simulink library "PowerFlowLib"  (Simulink 8.1)
settings: Solver=ode45  StartTime=0.0  StopTime=10.0  RelTol=1e-3
undefined symbols (not defined in the file or in its folder): Air, AirProp, C, F1, F2, Fanmap, Fld1, Fld2, Fluid, fueltankdata, HydProp, HydraulicLoad, IBFD_exc, L, LoadFluidProps, magnitude, MSSN, n_alghts, PumpProp, pwr_alghts, R_fd_exc, Rcore, Ts, VBFD_exc
libraries: PowerFlowLib x35, simulink x19, powerlib_extras x2, dspstat3 x2
(part 7 of 12)

== system PowerFlowLib/Energy & Power Systems/Electrical/Loads/Constant Current Load ==
  I_rms : Inport
  P.F. : Inport  Port=2
  Vabc : Inport  Port=3
  Eta1 : Inport  Port=4
  Constant : Constant  Value=[0 -2*pi/3 2*pi/3]
  Demux : Demux  Outputs=3
  Fcn1 : Fcn  Expr=(u(1)<=1)*(1-u(1))
  Math Function : Math  Operator=square  SaturateOnIntegerOverflow=on
  Mean Value : powerlib_extras/Measurements/Mean Value  Period=1/60
  Product{,1..6} (7 alike) : Product  RndMeth=Zero
  Sqrt : Sqrt  SaturateOnIntegerOverflow=on
  Sum : Sum  Inputs=|+-
  Sum1 : Sum
  Trigonometric Function : Trigonometry  Operator=acos
  Trigonometric Function1 : Trigonometry
  Trigonometric Function2 : Trigonometry  Operator=atan2
  Trigonometric Function3 : Trigonometry  Operator=cos
  Trigonometric Function4 : Trigonometry
  abc to qd0 : Subsystem
  iabc : Outport
  P : Outport  Port=2
  P_loss1 : Outport  Port=3
  Q : Outport  Port=4
  wires:
  Math Function/1 -> Mean Value/1
  Mean Value/1 -> Sqrt/1
  Sqrt/1 -> Product4/2, Product6/2  "RMS"
  I_rms/1 -> Product/1, Product1/1
  P.F./1 -> Product/2, Trigonometric Function/1
  Trigonometric Function/1 -> Trigonometric Function1/1
  Trigonometric Function1/1 -> Product1/2
  Product/1 -> Product2/1, Product6/1
  Vabc/1 -> Demux/1
  Demux/1 -> abc to qd0/1(V_a), Math Function/1
  Demux/2 -> abc to qd0/2(V_b)
  Demux/3 -> abc to qd0/3(V_c)
  Trigonometric Function3/1 -> Product2/2
  Trigonometric Function4/1 -> Product3/2
  Trigonometric Function2/1 -> Sum/1
  Constant/1 -> Sum/2
  Sum/1 -> Trigonometric Function3/1, Trigonometric Function4/1
  Product2/1 -> Sum1/1
  Product3/1 -> Sum1/2
  Sum1/1 -> iabc/1
  abc to qd0/2(V_d) -> Trigonometric Function2/1
  abc to qd0/1(V_q) -> Trigonometric Function2/2
  Product1/1 -> Product3/1, Product4/1
  Eta1/1 -> Fcn1/1
  Product5/1 -> P_loss1/1
  Product6/1 -> P/1, Product5/1
  Product4/1 -> Q/1
  Fcn1/1 -> Product5/2

== system PowerFlowLib/Energy & Power Systems/Electrical/Loads/Constant Power Load ==
  S : Inport
  P.F. : Inport  Port=2
  Vabc : Inport  Port=3
  Eta : Inport  Port=4
  Constant : Constant  Value=[0 -2*pi/3 2*pi/3]
  Demux : Demux  Outputs=3
  Fcn : Fcn  Expr=u(1)/(u(3)+0.01)
  Fcn1 : Fcn  Expr=u(2)/(u(3)+0.01)
  Fcn2 : Fcn  Expr=(u(1)<=1)*(1-u(1))
  Math Function : Math  Operator=square  SaturateOnIntegerOverflow=on
  Mean Value : powerlib_extras/Measurements/Mean Value  Period=1/60
  Mux : Mux  Inputs=3
  Product{,1..4} (5 alike) : Product  RndMeth=Zero
  Scope : Scope
      settings: TimeRange=auto  MaxDataPoints=5000  SaveToWorkspace=off  SaveName=ScopeData  YMin=-10  YMax=10  SampleTime=-1
  Sqrt : Sqrt  SaturateOnIntegerOverflow=on
  Sum : Sum  Inputs=|+-
  Sum1 : Sum
  Trigonometric Function : Trigonometry  Operator=acos
  Trigonometric Function1 : Trigonometry
  Trigonometric Function2 : Trigonometry  Operator=atan2
  Trigonometric Function3 : Trigonometry  Operator=cos
  Trigonometric Function4 : Trigonometry
  abc to qd0 : Subsystem
  iabc : Outport
  P : Outport  Port=2
  Q : Outport  Port=3
  P_loss : Outport  Port=4
  wires:
  Math Function/1 -> Mean Value/1
  Mean Value/1 -> Sqrt/1
  Sqrt/1 -> Scope/1, Mux/3  "RMS"
  S/1 -> Product/1, Product1/1
  P.F./1 -> Product/2, Trigonometric Function/1
  Trigonometric Function/1 -> Trigonometric Function1/1
  Trigonometric Function1/1 -> Product1/2
  Product/1 -> Mux/1, P/1, Product4/1
  Product1/1 -> Mux/2, Q/1
  Mux/1 -> Fcn/1, Fcn1/1
  Vabc/1 -> Demux/1
  Demux/1 -> abc to qd0/1(V_a), Math Function/1
  Demux/2 -> abc to qd0/2(V_b)
  Demux/3 -> abc to qd0/3(V_c)
  Fcn/1 -> Product2/1
  Fcn1/1 -> Product3/1
  Trigonometric Function3/1 -> Product2/2
  Trigonometric Function4/1 -> Product3/2
  Trigonometric Function2/1 -> Sum/1
  Constant/1 -> Sum/2
  Sum/1 -> Trigonometric Function3/1, Trigonometric Function4/1
  Product2/1 -> Sum1/1
  Product3/1 -> Sum1/2
  Sum1/1 -> iabc/1
  abc to qd0/2(V_d) -> Trigonometric Function2/1
  abc to qd0/1(V_q) -> Trigonometric Function2/2
  Eta/1 -> Fcn2/1
  Product4/1 -> P_loss/1
  Fcn2/1 -> Product4/2

== system PowerFlowLib/Energy & Power Systems/Electrical/Loads/Enabled  DC Load1 ==
  VDC : Inport
  Control : Inport  Port=2
  Enable : EnablePort
  Demux : Demux  Outputs=2
  Fcn1 : Fcn  Expr=u(1)/(u(2)+0.01)
  Mux : Mux  Inputs=2
  Sum : Sum
  iDC : Outport
  wires:
  Demux/2 -> Mux/1
  Mux/1 -> Fcn1/1
  Fcn1/1 -> Sum/2
  VDC/1 -> Mux/2
  Sum/1 -> iDC/1
  Demux/1 -> Sum/1
  Control/1 -> Demux/1

== system PowerFlowLib/Energy & Power Systems/Electrical/Loads/Enabled_AC_Loadloss ==
  Load Master Vector : Inport
  Vdq0 : Inport  Port=2
  Enable : EnablePort
  Enabled Subsystem : Subsystem  TreatAsAtomicUnit=on
  Enabled Subsystem1 : Subsystem  TreatAsAtomicUnit=on
  Sum1 : Sum  Inputs=|++
  Idq0 : Outport
  loss : Outport  Port=2
  wires:
  Vdq0/1 -> Enabled Subsystem/1("Vdq0 "), Enabled Subsystem1/1("Vdq0 ")
  Enabled Subsystem1/1(Idq0) -> Sum1/1
  Enabled Subsystem/1(Idq0) -> Sum1/2
  Sum1/1 -> Idq0/1
  Load Master Vector/1 -> Enabled Subsystem1/2(Ext vector)
  Enabled Subsystem/2(loss) -> loss/1

== system PowerFlowLib/Energy & Power Systems/Electrical/Loss Estimation/DC/DC Converter - Boost ==
  Input current : Inport
  Diode drop : Inport  Port=2
  Switch drop : Inport  Port=3
  "ESR (C) " : Inport  Port=4
  Cap Current  (Iin-Iout) : Inport  Port=5
  ESR (L) : Inport  Port=6
  d(t) : Inport  Port=7
  Add : Sum
  Add1 : Sum
  Add2 : Sum  Inputs=+-
  Add3 : Sum
  Constant : Constant
  Math Function : Math  Operator=square  SaturateOnIntegerOverflow=on
  Math Function1 : Math  Operator=square  SaturateOnIntegerOverflow=on
  Product : Product  Inputs=3  RndMeth=Zero
  Product1 : Product  RndMeth=Zero
  Product2 : Product  RndMeth=Zero
  Product3 : Product  Inputs=3  RndMeth=Zero
  Total Loss : Outport
  Conduction Loss : Outport  Port=2
  Parasitic Loss : Outport  Port=3
  wires:
  Switch drop/1 -> Product/1
  Input current/1 -> Math Function1/1, Product/2, Product3/1
  Math Function/1 -> Product1/1
  "ESR (C) "/1 -> Product1/2
  Add/1 -> Total Loss/1
  Cap Current  (Iin-Iout)/1 -> Math Function/1
  Math Function1/1 -> Product2/1
  ESR (L)/1 -> Product2/2
  Product1/1 -> Add1/1
  Product2/1 -> Add1/2
  Add1/1 -> Parasitic Loss/1, Add/2
  Constant/1 -> Add2/1
  Diode drop/1 -> Product3/3
  Add2/1 -> Product3/2
  d(t)/1 -> Add2/2, Product/3
  Product3/1 -> Add3/2
  Add3/1 -> Conduction Loss/1, Add/1
  Product/1 -> Add3/1

== system PowerFlowLib/Energy & Power Systems/Electrical/Loss Estimation/DC/DC Converter - Buck ==
  Input current : Inport
  Diode Drop : Inport  Port=2
  Switch drop : Inport  Port=3
  "ESR (C) " : Inport  Port=4
  Cap Current  (Iin-Iout) : Inport  Port=5
  ESR (L) : Inport  Port=6
  d(t) : Inport  Port=7
  Add : Sum
  Add1 : Sum
  Add2 : Sum  Inputs=+-
  Add3 : Sum
  Constant : Constant
  Math Function : Math  Operator=square  SaturateOnIntegerOverflow=on
  Math Function1 : Math  Operator=square  SaturateOnIntegerOverflow=on
  Product : Product  Inputs=3  RndMeth=Zero
  Product1 : Product  RndMeth=Zero
  Product2 : Product  RndMeth=Zero
  Product3 : Product  Inputs=3  RndMeth=Zero
  Total Loss : Outport
  Conduction Loss : Outport  Port=2
  Parasitic Loss : Outport  Port=3
  wires:
  Add1/1 -> Add/2, Parasitic Loss/1
  Product2/1 -> Add1/2
  Product1/1 -> Add1/1
  ESR (L)/1 -> Product2/2
  Math Function1/1 -> Product2/1
  Cap Current  (Iin-Iout)/1 -> Math Function/1
  Add/1 -> Total Loss/1
  "ESR (C) "/1 -> Product1/2
  Math Function/1 -> Product1/1
  Input current/1 -> Math Function1/1, Product/2, Product3/1
  Switch drop/1 -> Product/1
  Product/1 -> Add/1, Add3/1
  d(t)/1 -> Add2/2, Product/3
  Diode Drop/1 -> Product3/3
  Constant/1 -> Add2/1
  Add2/1 -> Product3/2
  Product3/1 -> Add3/2
  Add3/1 -> Conduction Loss/1

== system PowerFlowLib/Energy & Power Systems/Electrical/Loss Estimation/Three-Phase ACTIVE RECTIFIER ==
  Vdc : Inport
  Trise : Inport  Port=2
  Tfall : Inport  Port=3
  Rectifier Line current : Inport  Port=4
  H- Band : Inport  Port=5
  Source Ls : Inport  Port=6
  Source Vol (RMS) : Inport  Port=7
  Line Frequency : Inport  Port=8
  VCE drop : Inport  Port=9
  Add : Sum
  Integrator : Integrator
  No. of IGBT switches : Gain  Gain=6
  "No. of series vol drops " : Gain  Gain=2
  Product : Product  RndMeth=Zero
  Switch Loss : Subsystem
  Switching Frequency : Subsystem
  Total Loss : Outport
  Switching Loss : Outport  Port=2
  Conduction Loss : Outport  Port=3
  Inst Fsw : Outport  Port=4
  Mean Fsw : Outport  Port=5
  wires:
  Add/1 -> Total Loss/1
  No. of IGBT switches/1 -> Switching Loss/1, Add/1
  Product/1 -> Conduction Loss/1, Add/2
  "No. of series vol drops "/1 -> Product/2
  VCE drop/1 -> "No. of series vol drops "/1
  Switching Frequency/2(Mean fsw) -> Mean Fsw/1, Switch Loss/5(Fsw mean)
  Line Frequency/1 -> Integrator/1
  Vdc/1 -> Switch Loss/1(Vdc), Switching Frequency/1(Vdc)
  Source Vol (RMS)/1 -> Switching Frequency/2(Source Vol (RMS))
  Source Ls/1 -> Switching Frequency/4(Lls)
  Integrator/1 -> Switching Frequency/5(theta)
  Switching Frequency/1(Inst. fsw) -> Inst Fsw/1
  Trise/1 -> Switch Loss/2(Trise)
  Tfall/1 -> Switch Loss/3(Tfall)
  Rectifier Line current/1 -> Product/1, Switch Loss/4(Inverter Phae current)
  H- Band/1 -> Switching Frequency/3(H-Band)
  Switch Loss/1(Switching Loss) -> No. of IGBT switches/1

== system PowerFlowLib/Energy & Power Systems/Electrical/Loss Estimation/Three-Phase Diode Full Bridge  PASSIVE RECTIFIER ==
  AC line current : Inport
  Diode drop : Inport  Port=2
  "ESR (C) " : Inport  Port=3
  Cap Current  (Iin-Iout) : Inport  Port=4
  ESR (L) : Inport  Port=5
  Add : Sum
  Add1 : Sum
  Math Function : Math  Operator=square  SaturateOnIntegerOverflow=on
  Math Function1 : Math  Operator=square  SaturateOnIntegerOverflow=on
  No. of  series diodes : Gain  Gain=2
  Product : Product  RndMeth=Zero
  Product1 : Product  RndMeth=Zero
  Product2 : Product  RndMeth=Zero
  Total Loss : Outport
  Conduction Loss : Outport  Port=2
  Parasitic Loss : Outport  Port=3
  wires:
  No. of  series diodes/1 -> Conduction Loss/1, Add/1
  Diode drop/1 -> Product/1
  AC line current/1 -> Product/2, Math Function1/1
  Product/1 -> No. of  series diodes/1
  Math Function/1 -> Product1/1
  "ESR (C) "/1 -> Product1/2
  Add/1 -> Total Loss/1
  Cap Current  (Iin-Iout)/1 -> Math Function/1
  Math Function1/1 -> Product2/1
  ESR (L)/1 -> Product2/2
  Product1/1 -> Add1/1
  Product2/1 -> Add1/2
  Add1/1 -> Parasitic Loss/1, Add/2

== system PowerFlowLib/Energy & Power Systems/Electrical/Loss Estimation/Three-Phase Full Bridge Inverter CONSTANT FREQUENCY ==
  Vdc : Inport
  Trise : Inport  Port=2
  Tfall : Inport  Port=3
  Inverter Phase current : Inport  Port=4
  PWM frequency : Inport  Port=5
  VCE drop : Inport  Port=6
  Add : Sum
  No. of IGBT switches : Gain  Gain=6
  "No. of series vol drops " : Gain  Gain=3
  Product : Product  RndMeth=Zero
  Switch Loss : Subsystem
  Total Loss : Outport
  Switching Loss : Outport  Port=2
  Conduction Loss : Outport  Port=3
  wires:
  Trise/1 -> Switch Loss/2(Trise)
  Tfall/1 -> Switch Loss/3(Tfall)
  Inverter Phase current/1 -> Switch Loss/4(Inverter phase current), Product/1
  Switch Loss/1(Switch Loss) -> No. of IGBT switches/1
  PWM frequency/1 -> Switch Loss/5(Fsw mean)
  Vdc/1 -> Switch Loss/1(Vdc)
  VCE drop/1 -> "No. of series vol drops "/1
  "No. of series vol drops "/1 -> Product/2
  Add/1 -> Total Loss/1
  No. of IGBT switches/1 -> Add/1, Switching Loss/1
  Product/1 -> Add/2, Conduction Loss/1

== system PowerFlowLib/Energy & Power Systems/Electrical/Loss Estimation/Three-Phase Full Bridge Inverter VARIABLE FREQUENCY ==
  Vdc : Inport
  Trise : Inport  Port=2
  Tfall : Inport  Port=3
  Inverter phase current : Inport  Port=4
  H- Band : Inport  Port=5
  Series Ls : Inport  Port=6
  Back Vol (RMS) : Inport  Port=7
  Line Frequency : Inport  Port=8
  VCE drop : Inport  Port=9
  Add : Sum
  Integrator : Integrator
  No. of IGBT switches : Gain  Gain=6
  "No. of series vol drops " : Gain  Gain=3
  Product : Product  RndMeth=Zero
  Switch Loss : Subsystem
  Switching Frequency : Subsystem
  Total Loss : Outport
  Switching Loss : Outport  Port=2
  Conduction Loss : Outport  Port=3
  Inst Fsw : Outport  Port=4
  Mean Fsw : Outport  Port=5
  wires:
  Switch Loss/1(Switching Loss) -> No. of IGBT switches/1
  H- Band/1 -> Switching Frequency/3(H-Band)
  Inverter phase current/1 -> Switch Loss/4(Inverter Phae current), Product/1
  Tfall/1 -> Switch Loss/3(Tfall)
  Trise/1 -> Switch Loss/2(Trise)
  Switching Frequency/1(Inst. fsw) -> Inst Fsw/1
  Integrator/1 -> Switching Frequency/5(theta)
  Series Ls/1 -> Switching Frequency/4(Lls)
  Back Vol (RMS)/1 -> Switching Frequency/2(Machine vol (RMS))
  Vdc/1 -> Switching Frequency/1(Vdc), Switch Loss/1(Vdc)
  Line Frequency/1 -> Integrator/1
  Switching Frequency/2(Mean fsw) -> Switch Loss/5(Fsw mean), Mean Fsw/1
  VCE drop/1 -> "No. of series vol drops "/1
  "No. of series vol drops "/1 -> Product/2
  Product/1 -> Add/2, Conduction Loss/1
  No. of IGBT switches/1 -> Add/1, Switching Loss/1
  Add/1 -> Total Loss/1

== system PowerFlowLib/Energy & Power Systems/Electrical/Machines/DC Position Servo ==
  T_load (Nm) : Inport
  theta* (degrees) : Inport  Port=2
  Constant2 : Constant  Value=Vf
  DC Machine : Subsystem
  Fcn : Fcn  Expr=u(1)/(u(2)+0.1)
  Gain : Gain
  Gain1 : Gain  Gain=Ki
  Gain3 : Gain  Gain=2
  Gain4 : Gain
  Gain5 : Gain  Gain=0
  Integrator : Integrator
  Integrator2 : Integrator
  Mux : Mux  Inputs=2
  Scope : Scope
      settings: TimeRange=auto  MaxDataPoints=5000  SaveToWorkspace=off  SaveName=ScopeData4  YMin=-0.005  YMax=-0.0005  SampleTime=-1
  Sum : Sum  Inputs=-++
  Sum1 : Sum  Inputs=|++
  Sum3 : Sum  Inputs=|-+
  w_m : Outport
  i_load : Outport  Port=2
  T_em : Outport  Port=3
  theta_m : Outport  Port=4
  Plosses : Outport  Port=5
  wires:
  DC Machine/5(Plosses) -> Plosses/1
  Sum/1 -> Gain/1, Integrator/1
  Integrator/1 -> Gain1/1
  Gain/1 -> Sum1/1
  Gain1/1 -> Sum1/2
  T_load (Nm)/1 -> DC Machine/3(Tload)
  DC Machine/6(Te) -> T_em/1
  Mux/1 -> Fcn/1
  DC Machine/3(Pe) -> Mux/1
  Constant2/1 -> DC Machine/1(Vf), Mux/2
  Fcn/1 -> i_load/1
  Sum3/1 -> Gain4/1, Integrator2/1
  Integrator2/1 -> Gain5/1
  DC Machine/2(Ia) -> Scope/1
  DC Machine/8(theta) -> Sum3/1, theta_m/1
  theta* (degrees)/1 -> Sum3/2
  Gain4/1 -> Sum/2
  Gain5/1 -> Sum/3
  Sum1/1 -> DC Machine/2(Va)
  DC Machine/7(Speed) -> w_m/1, Gain3/1
  Gain3/1 -> Sum/1

== system PowerFlowLib/Energy & Power Systems/Electrical/Machines/DC Speed Servo ==
  T_load (Nm) : Inport
  Speed_ref (RPM) : Inport  Port=2
  DC Machine : Subsystem
  Fcn : Fcn  Expr=u(1)/(u(2)+0.1)
  Gain2 : Gain  Gain=60/(2*pi)
  Mux : Mux  Inputs=2
  PID Controller : simulink/Continuous/PID Controller  Controller=PID  TimeDomain=Continuous-time  SampleTime=-1  IntegratorMethod=Forward Euler  FilterMethod=Forward Euler  Form=Parallel  UseFilter=on  ControllerParametersSource=internal  P=1  I=0.1  D=0  N=100  InitialConditionSource=internal  InitialConditionForIntegrator=0  InitialConditionForFilter=0  ExternalReset=none  LimitOutput=off  UpperSaturationLimit=inf  LowerSaturationLimit=-inf  LinearizeAsGain=on  AntiWindupMode=none  Kb=1  TrackingMode=off  Kt=1  PParamMin=[]  PParamMax=[]  IParamMin=[]  IParamMax=[]  DParamMin=[]  DParamMax=[]  NParamMin=[]  NParamMax=[]  KbParamMin=[]  KbParamMax=[]  KtParamMin=[]  KtParamMax=[]  POutMin=[]  POutMax=[]  IOutMin=[]  IOutMax=[]  DOutMin=[]  DOutMax=[]  NOutMin=[]  NOutMax=[]  KbOutMin=[]  KbOutMax=[]  KtOutMin=[]  KtOutMax=[]  IntegratorOutMin=[]  IntegratorOutMax=[]  FilterOutMin=[]  FilterOutMax=[]  SumOutMin=[]  SumOutMax=[]  SumI1OutMin=[]  SumI1OutMax=[]  SumI2OutMin=[]  SumI2OutMax=[]  SumI3OutMin=[]  SumI3OutMax=[]  SumDOutMin=[]  SumDOutMax=[]  SaturationOutMin=[]  SaturationOutMax=[]  IntegratorContinuousStateAttributes=''  IntegratorStateMustResolveToSignalObject=off  IntegratorRTWStateStorageClass=Auto  FilterContinuousStateAttributes=''  FilterStateMustResolveToSignalObject=off  FilterRTWStateStorageClass=Auto  DifferentiatorICPrevScaledInput=0  DifferentiatorOutMin=[]  DifferentiatorOutMax=[]
  Speed Reference1 : Constant  Value=Vf
  Sum : Sum  Inputs=-+|
  w_m : Outport
  i_load : Outport  Port=2
  T_em : Outport  Port=3
  Ploss : Outport  Port=4
  wires:
  PID Controller/1 -> DC Machine/2(Va)
  Speed Reference1/1 -> Mux/2, DC Machine/1(Vf)
  DC Machine/7(Speed) -> Gain2/1
  Fcn/1 -> i_load/1
  DC Machine/3(Pe) -> Mux/1
  Mux/1 -> Fcn/1
  DC Machine/6(Te) -> T_em/1
  T_load (Nm)/1 -> DC Machine/3(Tload)
  Speed_ref (RPM)/1 -> Sum/2
  Gain2/1 -> w_m/1, Sum/1
  Sum/1 -> PID Controller/1
  DC Machine/5(Plosses) -> Ploss/1

== system PowerFlowLib/Energy & Power Systems/Electrical/Machines/Induction motor ==
  note: Implement Core Loss
  vqs : Inport
  vds : Inport  Port=2
  v0s : Inport  Port=3
  wr_mech : Inport  Port=4
  Cooing fan torque : Lookup  InputValues=IM_fan_omega  Table=IM_fan_torque  SaturateOnIntegerOverflow=on
  D-axis block : Subsystem
  Electric torque : Fcn  Expr=3/4*IM_Poles/IM_wb*(u[3]*u[2]-u[1]*u[4])
  Mux : Mux
  Mux1 : Mux  Inputs=3
  Mux2 : Mux  Inputs=3
  P/2 : Gain  Gain=IM_Poles/2  SaturateOnIntegerOverflow=on  OutDataTypeStr=Inherit: Same as input  ParamDataTypeStr=Inherit: Same as input
  Power Loss Measurement : Subsystem
  Product : Product  SaturateOnIntegerOverflow=on  InputSameDT=on  OutDataTypeStr=Inherit: Same as first input
  Product1 : Product  SaturateOnIntegerOverflow=on  InputSameDT=on  OutDataTypeStr=Inherit: Same as first input
  Q-axis block : Subsystem
  Sum : Sum  Inputs=+-  SaturateOnIntegerOverflow=on  InputSameDT=on  OutDataTypeStr=Inherit: Same as first input
  Sum1 : Sum  Inputs=+-  SaturateOnIntegerOverflow=on  InputSameDT=on  OutDataTypeStr=Inherit: Same as first input
  i_0s : Integrator
  rs : Gain  Gain=IM_rs  SaturateOnIntegerOverflow=on  OutDataTypeStr=Inherit: Same as input  ParamDataTypeStr=Inherit: Same as input
  wb/Xls : Gain  Gain=IM_wb/IM_Xls  SaturateOnIntegerOverflow=on  OutDataTypeStr=Inherit: Same as input  ParamDataTypeStr=Inherit: Same as input
  T_em : Outport
  iqs : Outport  Port=2
  ids : Outport  Port=3
  i0s : Outport  Port=4
  wires:
  Cooing fan torque/1 -> Sum/2
  wr_mech/1 -> P/2/1, Cooing fan torque/1, [wr_mech]
  P/2/1 -> Product1/2, Product/1
  Electric torque/1 -> Sum/1
  D-axis block/2(ids) -> Mux/4, ids/1, [ids]
  Q-axis block/2(iqs) -> Mux/2, iqs/1, [iqs]
  i_0s/1 -> rs/1, i0s/1, [i0s]
  rs/1 -> Sum1/2
  wb/Xls/1 -> i_0s/1
  Sum1/1 -> wb/Xls/1
  v0s/1 -> Sum1/1, [v0s]
  Sum/1 -> T_em/1, [T_em]
  Mux/1 -> Electric torque/1
  D-axis block/1(pds) -> Mux/3, [pds]
  Q-axis block/1(pqs) -> Mux/1, [pqs]
  vds/1 -> D-axis block/1(vds), [vds]
  vqs/1 -> Q-axis block/1(vqs), [vqs]
  D-axis block/3(pdr) -> Product/2
  Q-axis block/3(pqr) -> Product1/1
  Product1/1 -> D-axis block/2(wr*pqr)
  Product/1 -> Q-axis block/2(wr*pdr)
  Mux1/1 -> Power Loss Measurement/1(vqd0s)
  [vqs] -> Mux1/1
  [vds] -> Mux1/2
  [v0s] -> Mux1/3
  [iqs] -> Mux2/1
  [ids] -> Mux2/2
  [i0s] -> Mux2/3
  Mux2/1 -> Power Loss Measurement/2(iqd0s)
  [T_em] -> Power Loss Measurement/3(T_em)
  [wr_mech] -> Power Loss Measurement/4(wr_mech)
  Power Loss Measurement/1(P_el) -> [P_el]
  Power Loss Measurement/2(P_m) -> [P_m]
  Power Loss Measurement/3(P_loss) -> [P_loss]

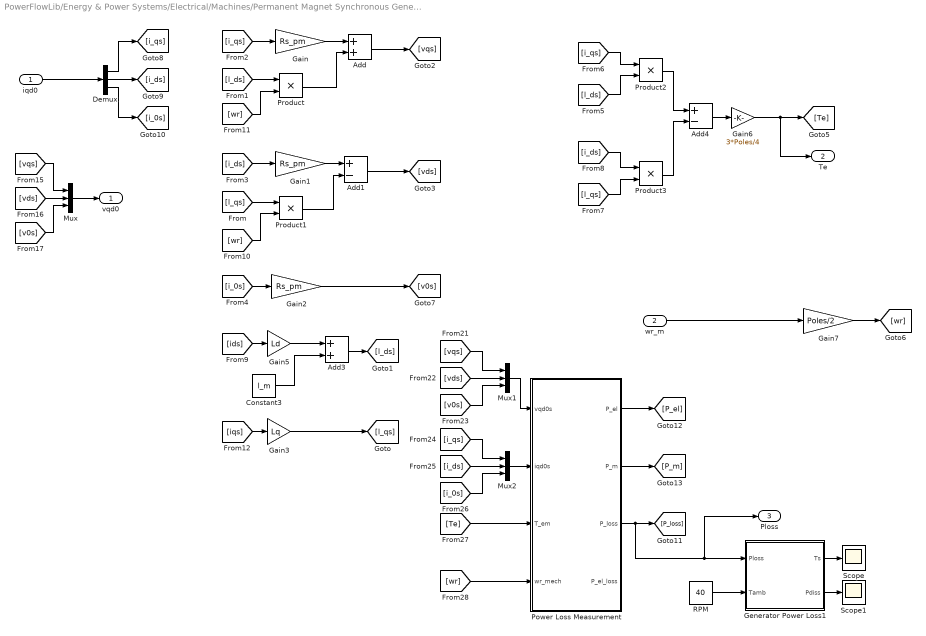
== system PowerFlowLib/Energy & Power Systems/Electrical/Machines/Permanent Magnet Synchronous Generator1 ==
  iqd0 : Inport
  wr_m : Inport  Port=2
  Add : Sum
  Add1 : Sum  Inputs=+-
  Add3 : Sum
  Add4 : Sum  Inputs=+-
  Constant3 : Constant  Value=l_m
  Demux : Demux  Outputs=3
  Gain : Gain  Gain=Rs_pm
  Gain1 : Gain  Gain=Rs_pm
  Gain2 : Gain  Gain=Rs_pm
  Gain3 : Gain  Gain=Lq
  Gain5 : Gain  Gain=Ld
  Gain6 : Gain  Gain=3*Poles/4
  Gain7 : Gain  Gain=Poles/2
  Generator Power Loss1 : Subsystem
  Mux : Mux  Inputs=3
  Mux1 : Mux  Inputs=3
  Mux2 : Mux  Inputs=3
  Power Loss Measurement : Subsystem
  Product{,1..3} (4 alike) : Product  RndMeth=Zero
  RPM : Constant  Value=40
  Scope : Scope
      settings: TimeRange=auto  MaxDataPoints=5000  SaveToWorkspace=off  SaveName=ScopeData10  YMin=40  YMax=100  SampleTime=-1
  Scope1 : Scope
      settings: TimeRange=auto  MaxDataPoints=5000  SaveToWorkspace=off  SaveName=ScopeData11  YMin=-10  YMax=10  SampleTime=-1
  vqd0 : Outport
  Te : Outport  Port=2
  Ploss : Outport  Port=3
  wires:
  Generator Power Loss1/2(Pdiss) -> Scope1/1
  Generator Power Loss1/1(Ts) -> Scope/1
  RPM/1 -> Generator Power Loss1/2(Tamb)
  Gain6/1 -> [Te], Te/1
  wr_m/1 -> Gain7/1
  Mux1/1 -> Power Loss Measurement/1(vqd0s)
  [vqs] -> Mux1/1
  [vds] -> Mux1/2
  [v0s] -> Mux1/3
  [i_qs] -> Mux2/1
  [i_ds] -> Mux2/2
  [i_0s] -> Mux2/3
  Mux2/1 -> Power Loss Measurement/2(iqd0s)
  [Te] -> Power Loss Measurement/3(T_em)
  [wr] -> Power Loss Measurement/4(wr_mech)
  Power Loss Measurement/1(P_el) -> [P_el]
  Power Loss Measurement/2(P_m) -> [P_m]
  Power Loss Measurement/3(P_loss) -> Ploss/1, Generator Power Loss1/1(Ploss), [P_loss]
  Demux/3 -> [i_0s]
  Demux/2 -> [i_ds]
  Demux/1 -> [i_qs]
  Mux/1 -> vqd0/1
  [v0s] -> Mux/3
  [vds] -> Mux/2
  [vqs] -> Mux/1
  Add4/1 -> Gain6/1
  Product3/1 -> Add4/2
  Product2/1 -> Add4/1
  [l_qs] -> Product3/2
  [i_ds] -> Product3/1
  [l_ds] -> Product2/2
  [i_qs] -> Product2/1
  Gain7/1 -> [wr]
  iqd0/1 -> Demux/1
  [i_0s] -> Gain2/1
  Gain2/1 -> [v0s]
  [i_qs] -> Gain/1
  [l_ds] -> Product/1
  [wr] -> Product/2
  [i_ds] -> Gain1/1
  [l_qs] -> Product1/1
  Add3/1 -> [l_ds]
  Constant3/1 -> Add3/2
  [wr] -> Product1/2
  Gain/1 -> Add/1
  Product/1 -> Add/2
  Gain1/1 -> Add1/1
  Product1/1 -> Add1/2
  Add/1 -> [vqs]
  Add1/1 -> [vds]
  [ids] -> Gain5/1
  Gain5/1 -> Add3/1
  [iqs] -> Gain3/1
  Gain3/1 -> [l_qs]

== system PowerFlowLib/Energy & Power Systems/Electrical/Machines/Synchronous Machine P.U. dq0 ==
  note: Dynamic model of P.U. Synchronous Generators v1.0
      | Base frequency is 60 Hz
      | Network transients are omitted
      | by Tutku Buyukdegirmenci
  note: Core Dynaimcs
  note: Outputs
  note: Inputs
  note: 0 axis to be implemented
  idq0 : Inport
  w : Inport  Port=2
  ifd : Inport  Port=3
  Demux : Demux  Outputs=3
  Dynamics : Subsystem
  Electromagnetic Torque Output Power : Subsystem
  Gain1 : Gain  Gain=Xmd/R_fd/VBFD
  Gain2 : Gain  Gain=1/wB
  Gain3 : Gain  Gain=R_fd/VBFD*IBFD
  Gain4 : Gain  Gain=P/2
  Generator Power Loss : Subsystem
  Generator Power Loss1 : Subsystem
  Memory1 : Memory  InheritSampleTime=on
  Mux : Mux  Inputs=3
  RPM : Constant  Value=40
  Scope : Scope
      settings: TimeRange=auto  MaxDataPoints=5000  SaveToWorkspace=off  SaveName=ScopeData8  YMin=40  YMax=100  SampleTime=-1
  Scope1 : Scope
      settings: TimeRange=auto  MaxDataPoints=5000  SaveToWorkspace=off  SaveName=ScopeData9  YMin=-10  YMax=10  SampleTime=-1
  Stator Voltage : Subsystem
  V0 : Constant  Value=0
  p.u. transform currents : Gain  Gain=1/IBDQ
  p.u. transform torque : Gain  Gain=TB
  p.u. transform voltages : Gain  Gain=VBDQ
  vdq0 : Outport
  Te : Outport  Port=2
  vfd : Outport  Port=3
  Ploss : Outport  Port=4
  wires:
  Generator Power Loss1/2(Pdiss) -> Scope1/1
  Generator Power Loss1/1(Ts) -> Scope/1
  RPM/1 -> Generator Power Loss1/2(Tamb)
  Gain4/1 -> Gain2/1
  [Efd] -> Dynamics/3(Efd)
  Memory1/1 -> vfd/1
  Gain3/1 -> Memory1/1, Gain1/1
  Gain1/1 -> [Efd]
  ifd/1 -> Gain3/1
  idq0/1 -> p.u. transform currents/1
  p.u. transform voltages/1 -> vdq0/1
  Generator Power Loss/3(PLOSS) -> Ploss/1, Generator Power Loss1/1(Ploss), [PLOSS]
  Generator Power Loss/2(PM) -> [PM]
  Generator Power Loss/1(PE) -> [PE]
  [Te] -> Generator Power Loss/5(Te)
  [nu] -> Generator Power Loss/6(w/ws)
  [Iq] -> Generator Power Loss/4(Iq)
  [Id] -> Generator Power Loss/3(Id)
  [Vq] -> Generator Power Loss/2(Eq)
  [Vd] -> Generator Power Loss/1(Ed)
  p.u. transform torque/1 -> Te/1
  p.u. transform currents/1 -> Demux/1
  [Te] -> p.u. transform torque/1
  Electromagnetic Torque Output Power/1(TE) -> [Te]
  [nu] -> Stator Voltage/7(w/ws)
  V0/1 -> Mux/3
  [Vq] -> Mux/2
  [Vd] -> Mux/1
  Mux/1 -> p.u. transform voltages/1
  [Iq] -> Electromagnetic Torque Output Power/2(Iq), Stator Voltage/2(Iq)
  [Id] -> Electromagnetic Torque Output Power/1(Id), Stator Voltage/1(Id)
  [Iq] -> Dynamics/2(Iq)
  [Id] -> Dynamics/1(Id)
  Gain2/1 -> [nu]
  Demux/2 -> [Iq]
  Demux/1 -> [Id]
  w/1 -> Gain4/1
  Stator Voltage/1(Ed) -> [Vd]
  Stator Voltage/2(Eq) -> [Vq]
  Dynamics/4(Phi_2q) -> Electromagnetic Torque Output Power/6(Phi_2q), Stator Voltage/6(Phi_2q)
  Dynamics/3(Phi_1d) -> Electromagnetic Torque Output Power/5(Phi_1d), Stator Voltage/5(Phi_1d)
  Dynamics/2(Ed1) -> Electromagnetic Torque Output Power/4(Ed1), Stator Voltage/4(Ed1)
  Dynamics/1(Eq1) -> Electromagnetic Torque Output Power/3(Eq1), Stator Voltage/3(Eq1)

== system PowerFlowLib/Energy & Power Systems/Electrical/Machines/Transformer ==
  Vin : Inport
  Iout : Inport  Port=2
  Gain : Gain  Gain=N2/N1
  Gain1 : Gain  Gain=N2/N1
  Gain2 : Gain  Gain=Rp
  Gain3 : Gain  Gain=Rs
  Memory : Memory  InheritSampleTime=on  LinearizeAsDelay=on
  Memory2 : Memory  InheritSampleTime=on  LinearizeAsDelay=on
  Sum1 : Sum  Inputs=|+-
  Sum2 : Sum  Inputs=|+-
  Vout : Outport
  Iin : Outport  Port=2
  wires:
  Vin/1 -> Sum1/1
  Iout/1 -> Gain1/1, Memory/1
  Gain1/1 -> Memory2/1
  Gain2/1 -> Sum1/2
  Sum1/1 -> Gain/1
  Gain/1 -> Sum2/1
  Sum2/1 -> Vout/1
  Memory/1 -> Gain3/1
  Memory2/1 -> Gain2/1, Iin/1
  Gain3/1 -> Sum2/2

== system PowerFlowLib/Energy & Power Systems/Electrical/Rectifiers/Single-phase Full Bridge Practical ==
  vin : Inport
  iout : Inport  Port=2
  1/C : Gain  Gain=1/C  SaturateOnIntegerOverflow=on  OutDataTypeStr=Inherit: Same as input  ParamDataTypeStr=Inherit: Same as input
  1/Rc : Gain  Gain=1/Rc  SaturateOnIntegerOverflow=on  OutDataTypeStr=Inherit: Same as input  ParamDataTypeStr=Inherit: Same as input
  Abs : Abs  SaturateOnIntegerOverflow=on
  Integrator : Integrator
  Product : Product  RndMeth=Zero
  Saturation : Saturate  UpperLimit=inf  LowerLimit=0
  Sign : Signum
  Sum : Sum  Inputs=+-  SaturateOnIntegerOverflow=on  InputSameDT=on  OutDataTypeStr=Inherit: Same as first input
  Sum1 : Sum  Inputs=+-  SaturateOnIntegerOverflow=on  InputSameDT=on  OutDataTypeStr=Inherit: Same as first input
  vout : Outport
  iin : Outport  Port=2
  wires:
  Product/1 -> iin/1
  Sign/1 -> Product/1
  vin/1 -> Sign/1, Abs/1
  Abs/1 -> Sum/1
  Saturation/1 -> Product/2, Sum1/1
  1/C/1 -> Integrator/1
  Sum1/1 -> 1/C/1
  Integrator/1 -> Sum/2, vout/1
  1/Rc/1 -> Saturation/1
  iout/1 -> Sum1/2
  Sum/1 -> 1/Rc/1

== system PowerFlowLib/Energy & Power Systems/Electrical/Rectifiers/Single-phase Half Bridge ==
  vin : Inport
  iout : Inport  Port=2
  1/C : Gain  Gain=1/C  SaturateOnIntegerOverflow=on  OutDataTypeStr=Inherit: Same as input  ParamDataTypeStr=Inherit: Same as input
  1/Rc : Gain  Gain=1/Rc  SaturateOnIntegerOverflow=on  OutDataTypeStr=Inherit: Same as input  ParamDataTypeStr=Inherit: Same as input
  Integrator : Integrator
  Saturation : Saturate  UpperLimit=inf  LowerLimit=0
  Saturation1 : Saturate  UpperLimit=inf  LowerLimit=0
  Sum : Sum  Inputs=+-  SaturateOnIntegerOverflow=on  InputSameDT=on  OutDataTypeStr=Inherit: Same as first input
  Sum1 : Sum  Inputs=+-  SaturateOnIntegerOverflow=on  InputSameDT=on  OutDataTypeStr=Inherit: Same as first input
  vout : Outport
  iin : Outport  Port=2
  wires:
  vin/1 -> Saturation1/1
  Saturation/1 -> iin/1, Sum1/1
  1/C/1 -> Integrator/1
  Sum1/1 -> 1/C/1
  Integrator/1 -> Sum/2, vout/1
  1/Rc/1 -> Saturation/1
  iout/1 -> Sum1/2
  Sum/1 -> 1/Rc/1
  Saturation1/1 -> Sum/1

== system PowerFlowLib/Energy & Power Systems/Electrical/Rectifiers/Three Phase Full Bridge Practical ==
  vin : Inport
  iout : Inport  Port=2
  1/C : Gain  Gain=1/C  SaturateOnIntegerOverflow=on  OutDataTypeStr=Inherit: Same as input  ParamDataTypeStr=Inherit: Same as input
  1/Rc : Gain  Gain=1/Rc  SaturateOnIntegerOverflow=on  OutDataTypeStr=Inherit: Same as input  ParamDataTypeStr=Inherit: Same as input
  Abs1 : Abs  SaturateOnIntegerOverflow=on
  Demux : Demux  Outputs=3
  Demux1 : Demux  Outputs=3
  Gain : Gain  Gain=[1 -1 0]
  Gain1 : Gain  Gain=[0 1 -1]
  Gain2 : Gain  Gain=[-1 0 1]
  Integrator : Integrator
  LL Calculation : Gain  Gain=[1 -1 0; 0 1 -1; -1 0 1]  Multiplication=Matrix(K*u)
  Logical Operator : Logic  IconShape=distinctive  AllPortsSameDT=off  OutDataTypeStr=float('double')
  Logical Operator1 : Logic  IconShape=distinctive  AllPortsSameDT=off  OutDataTypeStr=float('double')
  Logical Operator2 : Logic  IconShape=distinctive  AllPortsSameDT=off  OutDataTypeStr=float('double')
  MinMax : MinMax  Function=max
  Product{,1..3} (4 alike) : Product  RndMeth=Zero
  Relational Operator{,1..5} (6 alike) : RelationalOperator  OutDataTypeStr=boolean
  Saturation : Saturate  UpperLimit=inf  LowerLimit=0
  Scope2 : Scope  NumInputPorts=2
      settings: TimeRange=auto  MaxDataPoints=5000  SaveToWorkspace=off  SaveName=ScopeData3  YMin=-5~-5  YMax=5~5  SampleTime=-1
  Scope3 : Scope  NumInputPorts=2
      settings: TimeRange=auto  MaxDataPoints=5000  SaveToWorkspace=off  SaveName=ScopeData4  YMin=-5~-5  YMax=5~5  SampleTime=-1
  Sign : Signum
  Sign1 : Signum
  Sign2 : Signum
  Sum : Sum  Inputs=+-  SaturateOnIntegerOverflow=on  InputSameDT=on  OutDataTypeStr=Inherit: Same as first input
  Sum1 : Sum  Inputs=+-  SaturateOnIntegerOverflow=on  InputSameDT=on  OutDataTypeStr=Inherit: Same as first input
  Sum2 : Sum  Inputs=+++
  vout : Outport
  iin : Outport  Port=2
  wires:
  Saturation/1 -> Product/2, Sum1/1
  1/C/1 -> Integrator/1
  Sum1/1 -> 1/C/1
  Integrator/1 -> Sum/2, vout/1
  1/Rc/1 -> Saturation/1
  iout/1 -> Sum1/2
  Sum/1 -> 1/Rc/1
  MinMax/1 -> Sum/1
  vin/1 -> LL Calculation/1
  LL Calculation/1 -> Abs1/1, Scope2/2, Demux1/1
  Abs1/1 -> Demux/1, MinMax/1, Scope2/1
  Demux/1 -> Relational Operator3/2, Relational Operator5/2, Relational Operator/1, Relational Operator1/1
  Demux/2 -> Relational Operator/2, Relational Operator2/1, Relational Operator3/1, Relational Operator4/2
  Demux/3 -> Relational Operator1/2, Relational Operator2/2, Relational Operator4/1, Relational Operator5/1
  Relational Operator/1 -> Logical Operator/1
  Relational Operator1/1 -> Logical Operator/2
  Relational Operator2/1 -> Logical Operator1/1
  Relational Operator3/1 -> Logical Operator1/2
  Relational Operator4/1 -> Logical Operator2/1
  Relational Operator5/1 -> Logical Operator2/2
  Logical Operator/1 -> Gain/1, Scope3/1
  Logical Operator1/1 -> Gain1/1
  Logical Operator2/1 -> Gain2/1
  Sum2/1 -> Product/1
  Product/1 -> iin/1
  Gain/1 -> Product1/1
  Sign/1 -> Product1/2, Scope3/2
  Product1/1 -> Sum2/1
  Gain1/1 -> Product2/1
  Sign1/1 -> Product2/2
  Product2/1 -> Sum2/2
  Gain2/1 -> Product3/1
  Sign2/1 -> Product3/2
  Product3/1 -> Sum2/3
  Demux1/1 -> Sign/1
  Demux1/2 -> Sign1/1
  Demux1/3 -> Sign2/1

== system PowerFlowLib/Energy & Power Systems/Electrical/Rectifiers/Three-phase Full Bridge1 ==
  iout : Inport
  vin : Inport  Port=2
  1/C : Gain  Gain=1/C  SaturateOnIntegerOverflow=on  OutDataTypeStr=Inherit: Same as input  ParamDataTypeStr=Inherit: Same as input
  1/C1 : Gain  Gain=-1  SaturateOnIntegerOverflow=on  OutDataTypeStr=Inherit: Same as input  ParamDataTypeStr=Inherit: Same as input
  1/Rc : Gain  Gain=1/Rc  SaturateOnIntegerOverflow=on  OutDataTypeStr=Inherit: Same as input  ParamDataTypeStr=Inherit: Same as input
  Abs : Abs  SaturateOnIntegerOverflow=on
  Demux : Demux  Outputs=3
  Integrator : Integrator
  MinMax : MinMax  Function=max
  MinMax1 : MinMax  Function=max
  MinMax3 : MinMax
  Mux : Mux  Inputs=3
  Product : Product  RndMeth=Zero
  Relational Operator1 : RelationalOperator  Operator===  OutDataTypeStr=float('double')
  Relational Operator2 : RelationalOperator  Operator===  OutDataTypeStr=float('double')
  Saturation : Saturate  UpperLimit=inf  LowerLimit=0
  Sum{,1..4} (5 alike) : Sum  Inputs=+-  SaturateOnIntegerOverflow=on  InputSameDT=on  OutDataTypeStr=Inherit: Same as first input
  Sum8 : Sum  OutDataTypeStr=double  SaturateOnIntegerOverflow=on
  vout : Outport
  iin : Outport  Port=2
  wires:
  Sum8/1 -> Product/1
  1/C1/1 -> Sum8/2
  Relational Operator2/1 -> 1/C1/1
  Relational Operator1/1 -> Sum8/1
  MinMax3/1 -> Relational Operator2/1
  MinMax/1 -> Relational Operator1/1
  Sum4/1 -> Mux/3
  Sum3/1 -> Mux/2
  Sum2/1 -> Mux/1
  Demux/3 -> Sum4/1, Sum3/2
  Demux/2 -> Sum3/1, Sum2/2
  Demux/1 -> Sum4/2, Sum2/1
  Abs/1 -> MinMax1/1
  Mux/1 -> Abs/1
  MinMax1/1 -> Sum/1
  vin/1 -> Relational Operator2/2, MinMax3/1, Relational Operator1/2, MinMax/1, Demux/1
  Product/1 -> iin/1
  Sum/1 -> 1/Rc/1
  iout/1 -> Sum1/2
  1/Rc/1 -> Saturation/1
  Integrator/1 -> vout/1, Sum/2
  Sum1/1 -> 1/C/1
  1/C/1 -> Integrator/1
  Saturation/1 -> Product/2, Sum1/1

== system PowerFlowLib/Energy & Power Systems/Electrical/Rectifiers/three-phase  active rectifier ==
  qabc : Inport
  VRST : Inport  Port=2
  iLOAD : Inport  Port=3
  Gain : Gain  Gain=1/L
  Gain1 : Gain  Gain=1/C
  Gain2 : Gain  Gain=0.1
  Integrator : Integrator
  Integrator1 : Integrator
  Product : Product  SaturateOnIntegerOverflow=on  InputSameDT=on  OutDataTypeStr=Inherit: Same as first input
  Product1 : Product  SaturateOnIntegerOverflow=on  InputSameDT=on  OutDataTypeStr=Inherit: Same as first input
  Scope : Scope
      settings: TimeRange=0.08461538461538462  MaxDataPoints=5000  SaveToWorkspace=off  YMin=-9  YMax=9  SampleTime=-1
  Sum : Sum  Inputs=-+-
  Sum1 : Sum  Inputs=+
  Sum2 : Sum  Inputs=+-|
  Idc : Outport
  Vdc : Outport  Port=2
  wires:
  [VDC] -> Product/2
  Product/1 -> Sum/1
  Integrator/1 -> Product1/1, Scope/1, Gain2/1
  qabc/1 -> [qabc]
  [qabc] -> Product/1
  [qabc] -> Product1/2
  Product1/1 -> Sum1/1
  Sum1/1 -> Idc/1, Sum2/1
  VRST/1 -> Sum/2
  Sum/1 -> Gain/1
  Gain/1 -> Integrator/1
  iLOAD/1 -> Sum2/2
  Sum2/1 -> Gain1/1
  Gain1/1 -> Integrator1/1
  Integrator1/1 -> [VDC], Vdc/1
  Gain2/1 -> Sum/3

== system PowerFlowLib/Energy & Power Systems/Electrical/Rectifiers/three-phase  active rectifier Voltage Mode ==
  vqd0 : Inport
  cont : Inport  Port=2
  Vout : Inport  Port=3
  1/L : Gain  Gain=1/L  SaturateOnIntegerOverflow=on  OutDataTypeStr=Inherit: Same as input  ParamDataTypeStr=Inherit: Same as input
  Add : Sum  Inputs=+
  Demux : Demux  Outputs=3
  Mux : Mux  Inputs=3
  Product{,1..3} (4 alike) : Product  RndMeth=Zero
  Sqrt : Sqrt  SaturateOnIntegerOverflow=on
  Sum : Sum  Inputs=|+-
  Trigonometric Function : Trigonometry
  Trigonometric Function1 : Trigonometry  Operator=cos
  Trigonometric Function2 : Trigonometry  Operator=atan2
  iLstate : Integrator  LimitOutput=on  LowerSaturationLimit=0
  i_out : Outport
  iqd0 : Outport  Port=2
  wires:
  Vout/1 -> Sum/2
  vqd0/1 -> Demux/1, Product/1, Product/2
  Product/1 -> Add/1
  Add/1 -> Sqrt/1
  Sqrt/1 -> Product1/2
  cont/1 -> Product1/1
  Product1/1 -> Sum/1
  Trigonometric Function2/1 -> Trigonometric Function/1, Trigonometric Function1/1
  Trigonometric Function/1 -> Product2/1
  Trigonometric Function1/1 -> Product3/1
  Product2/1 -> Mux/1
  Product3/1 -> Mux/2
  Mux/1 -> iqd0/1
  Sum/1 -> 1/L/1
  1/L/1 -> iLstate/1
  iLstate/1 -> Product3/2, Product2/2, i_out/1
  Demux/1 -> Trigonometric Function2/1
  Demux/2 -> Trigonometric Function2/2

== system PowerFlowLib/Energy & Power Systems/Electrical/Systems/2 stage Boost converter (CCM Steady State) ==
  vin : Inport
  iout : Inport  Port=2
  vref : Inport  Port=3
  CHARGING CURRENT : Constant  Value=VREF1
  Fcn : Fcn  Expr=1-u
  Fcn1 : Fcn  Expr=1-u
  PID Controller : simulink/Continuous/PID Controller  Controller=PI  TimeDomain=Continuous-time  SampleTime=-1  IntegratorMethod=Forward Euler  FilterMethod=Forward Euler  Form=Parallel  UseFilter=on  ControllerParametersSource=internal  P=KP  I=KI  D=0  N=100  InitialConditionSource=internal  InitialConditionForIntegrator=0  InitialConditionForFilter=0  ExternalReset=none  LimitOutput=off  UpperSaturationLimit=inf  LowerSaturationLimit=-inf  LinearizeAsGain=off  AntiWindupMode=none  Kb=1  TrackingMode=off  Kt=1  PParamMin=[]  PParamMax=[]  IParamMin=[]  IParamMax=[]  DParamMin=[]  DParamMax=[]  NParamMin=[]  NParamMax=[]  KbParamMin=[]  KbParamMax=[]  KtParamMin=[]  KtParamMax=[]  POutMin=[]  POutMax=[]  IOutMin=[]  IOutMax=[]  DOutMin=[]  DOutMax=[]  NOutMin=[]  NOutMax=[]  KbOutMin=[]  KbOutMax=[]  KtOutMin=[]  KtOutMax=[]  IntegratorOutMin=[]  IntegratorOutMax=[]  FilterOutMin=[]  FilterOutMax=[]  SumOutMin=[]  SumOutMax=[]  SumI1OutMin=[]  SumI1OutMax=[]  SumI2OutMin=[]  SumI2OutMax=[]  SumI3OutMin=[]  SumI3OutMax=[]  SumDOutMin=[]  SumDOutMax=[]  SaturationOutMin=[]  SaturationOutMax=[]  IntegratorContinuousStateAttributes=''  IntegratorStateMustResolveToSignalObject=off  IntegratorRTWStateStorageClass=Auto  FilterContinuousStateAttributes=''  FilterStateMustResolveToSignalObject=off  FilterRTWStateStorageClass=Auto  DifferentiatorICPrevScaledInput=0  DifferentiatorOutMin=[]  DifferentiatorOutMax=[]
  PID Controller1 : simulink/Continuous/PID Controller  Controller=PI  TimeDomain=Continuous-time  SampleTime=-1  IntegratorMethod=Forward Euler  FilterMethod=Forward Euler  Form=Parallel  UseFilter=on  ControllerParametersSource=internal  P=KP  I=KI  D=0  N=100  InitialConditionSource=internal  InitialConditionForIntegrator=0  InitialConditionForFilter=0  ExternalReset=none  LimitOutput=off  UpperSaturationLimit=inf  LowerSaturationLimit=-inf  LinearizeAsGain=off  AntiWindupMode=none  Kb=1  TrackingMode=off  Kt=1  PParamMin=[]  PParamMax=[]  IParamMin=[]  IParamMax=[]  DParamMin=[]  DParamMax=[]  NParamMin=[]  NParamMax=[]  KbParamMin=[]  KbParamMax=[]  KtParamMin=[]  KtParamMax=[]  POutMin=[]  POutMax=[]  IOutMin=[]  IOutMax=[]  DOutMin=[]  DOutMax=[]  NOutMin=[]  NOutMax=[]  KbOutMin=[]  KbOutMax=[]  KtOutMin=[]  KtOutMax=[]  IntegratorOutMin=[]  IntegratorOutMax=[]  FilterOutMin=[]  FilterOutMax=[]  SumOutMin=[]  SumOutMax=[]  SumI1OutMin=[]  SumI1OutMax=[]  SumI2OutMin=[]  SumI2OutMax=[]  SumI3OutMin=[]  SumI3OutMax=[]  SumDOutMin=[]  SumDOutMax=[]  SaturationOutMin=[]  SaturationOutMax=[]  IntegratorContinuousStateAttributes=''  IntegratorStateMustResolveToSignalObject=off  IntegratorRTWStateStorageClass=Auto  FilterContinuousStateAttributes=''  FilterStateMustResolveToSignalObject=off  FilterRTWStateStorageClass=Auto  DifferentiatorICPrevScaledInput=0  DifferentiatorOutMin=[]  DifferentiatorOutMax=[]
  Product{,1..3} (4 alike) : Product  Inputs=*/  RndMeth=Zero
  Saturation : Saturate  UpperLimit=0.9  LowerLimit=0
  Saturation1 : Saturate  UpperLimit=0.9  LowerLimit=0
  Sum : Sum  Inputs=|+-
  Sum1 : Sum  Inputs=|+-
  vout : Outport
  duty1(t) : Outport  Port=2
  duty2(t) : Outport  Port=3
  iin : Outport  Port=4
  wires:
  Product1/1 -> iin/1
  PID Controller1/1 -> Saturation1/1
  Sum1/1 -> PID Controller1/1
  vref/1 -> Sum1/1
  Product3/1 -> Product1/1
  Product2/1 -> Sum1/2, vout/1
  iout/1 -> Product3/1
  Fcn1/1 -> duty2(t)/1, Product2/2, Product3/2
  Saturation1/1 -> Fcn1/1
  PID Controller/1 -> Saturation/1
  Sum/1 -> PID Controller/1
  CHARGING CURRENT/1 -> Sum/1
  Product/1 -> Product2/1, Sum/2
  Fcn/1 -> duty1(t)/1, Product/2, Product1/2
  vin/1 -> Product/1
  Saturation/1 -> Fcn/1

== system PowerFlowLib/Energy & Power Systems/Electrical/Systems/AC Service Bus ==
  Select : Inport
  sup_1 : Inport  Port=2
  sup_2 : Inport  Port=3
  sup_Load : Inport  Port=4
  Compare To Constant : simulink/Logic and Bit Operations/Compare To Constant  relop===  const=1  OutDataTypeStr=uint8
  Compare To Constant1 : simulink/Logic and Bit Operations/Compare To Constant  relop===  const=2  OutDataTypeStr=uint8
  Constant : Constant  Value=[0 0 0]
  Multiport Switch : MultiPortSwitch  Inputs=2
  Switch : Switch  Criteria=u2 ~= 0
  Switch1 : Switch  Criteria=u2 ~= 0
  Vbus : Outport
  i_sup_1 : Outport  Port=2
  i_sup_2 : Outport  Port=3
  wires:
  Switch1/1 -> i_sup_2/1
  Switch/1 -> i_sup_1/1
  Constant/1 -> Switch1/3, Switch/3
  Compare To Constant1/1 -> Switch1/2
  Compare To Constant/1 -> Switch/2
  sup_Load/1 -> Switch1/1, Switch/1
  Select/1 -> Compare To Constant1/1, Compare To Constant/1, Multiport Switch/1
  sup_2/1 -> Multiport Switch/3
  sup_1/1 -> Multiport Switch/2
  Multiport Switch/1 -> Vbus/1

== system PowerFlowLib/Energy & Power Systems/Electrical/Systems/DC Service Bus ==
  Select : Inport
  sup_1 : Inport  Port=2
  sup_2 : Inport  Port=3
  sup_Load : Inport  Port=4
  sup_charge : Inport  Port=5
  Compare To Constant : simulink/Logic and Bit Operations/Compare To Constant  relop===  const=1  OutDataTypeStr=uint8
  Compare To Constant1 : simulink/Logic and Bit Operations/Compare To Constant  relop===  const=2  OutDataTypeStr=uint8
  Constant : Constant  Value=[0]
  Multiport Switch : MultiPortSwitch  Inputs=2
  Sum : Sum  Inputs=|+-
  Switch : Switch  Criteria=u2 ~= 0
  Switch1 : Switch  Criteria=u2 ~= 0
  Vbus : Outport
  i_sup_1 : Outport  Port=2
  i_sup_2 : Outport  Port=3
  wires:
  Switch1/1 -> i_sup_2/1
  Switch/1 -> i_sup_1/1
  Constant/1 -> Switch1/3, Switch/3
  Compare To Constant1/1 -> Switch1/2
  Compare To Constant/1 -> Switch/2
  Select/1 -> Compare To Constant1/1, Compare To Constant/1, Multiport Switch/1
  sup_2/1 -> Multiport Switch/3
  sup_1/1 -> Multiport Switch/2
  Multiport Switch/1 -> Vbus/1
  sup_Load/1 -> Sum/1
  sup_charge/1 -> Sum/2
  Sum/1 -> Switch/1, Switch1/1

== system PowerFlowLib/Energy & Power Systems/Electrical/Systems/GND Service Bus ==
  iout : Inport
  Constant : Constant  Value=[120*sqrt(2) 0 0]
  vout : Outport
  wires:
  Constant/1 -> vout/1
  iout/1 -> ?

== system PowerFlowLib/Energy & Power Systems/Electrical/Systems/Gearbox ==
  w_engine : Inport
  T_gen : Inport  Port=2
  1-tran_efficiency : Gain  Gain=1-Gear_Efficiency/100  SaturateOnIntegerOverflow=on  OutDataTypeStr=Inherit: Same as input  ParamDataTypeStr=Inherit: Same as input
  Gain : Gain  Gain=Gear_Ratio
  Gain1 : Gain  Gain=Gear_Ratio
  Memory : Memory
  Memory1 : Memory
  Sum : Sum  Inputs=-++  SaturateOnIntegerOverflow=on  InputSameDT=on  OutDataTypeStr=Inherit: Same as first input
  gear1 NL loss : Lookup  InputValues=[0;1000;2000;3000;4000;5000;6000]*2*pi/60  Table=[0;0.735;1.334;1.491;1.525;1.212;1.276]  SaturateOnIntegerOverflow=on
  tran_efficiency : Gain  Gain=Gear_Efficiency/4/100  SaturateOnIntegerOverflow=on  OutDataTypeStr=Inherit: Same as input  ParamDataTypeStr=Inherit: Same as input
  w_shaft : Outport
  T_shaft : Outport  Port=2
  wires:
  Sum/1 -> T_shaft/1
  tran_efficiency/1 -> Sum/1
  1-tran_efficiency/1 -> Sum/2
  Memory1/1 -> Sum/3
  Gain/1 -> Memory/1
  gear1 NL loss/1 -> tran_efficiency/1
  w_engine/1 -> gear1 NL loss/1, Gain/1
  T_gen/1 -> 1-tran_efficiency/1, Gain1/1
  Gain1/1 -> Memory1/1
  Memory/1 -> w_shaft/1

== system PowerFlowLib/Energy & Power Systems/Electrical/Systems/Gen Bus w/ APU switch ==
  Select : Inport
  MAIN_Gen : Inport  Port=2
  APU_Gen : Inport  Port=3
  GND_sup : Inport  Port=4
  AUX_sup : Inport  Port=5
  i_Bus : Inport  Port=6
  Compare To Constant1 : simulink/Logic and Bit Operations/Compare To Constant  relop===  const=2  OutDataTypeStr=boolean
  Compare To Constant2 : simulink/Logic and Bit Operations/Compare To Constant  relop===  const=3  OutDataTypeStr=boolean
  Compare To Constant3 : simulink/Logic and Bit Operations/Compare To Constant  relop===  const=4  OutDataTypeStr=boolean
  Compare To Constant4 : simulink/Logic and Bit Operations/Compare To Constant  relop===  const=1  OutDataTypeStr=boolean
  Constant : Constant  Value=[0 0 0]
  Constant3 : Constant  Value=2
  Data Type Conversion : DataTypeConversion
  Logical Operator : Logic  Operator=NOT  AllPortsSameDT=off  OutDataTypeStr=boolean
  MATLAB Fcn : MATLABFcn  MATLABFcn=genwarning  OutputDimensions=1  SampleTime=bus_st
  Math Function : Math  Operator=square  SaturateOnIntegerOverflow=on
  Memory1 : Memory  X0=1
  Memory18 : Memory  InheritSampleTime=on
  Multiport Switch : MultiPortSwitch  Inputs=4
  Mux : Mux  Inputs=3
  Sqrt : Sqrt  SaturateOnIntegerOverflow=on
  Sum : Sum  Inputs=+
  Switch{,1..4} (5 alike) : Switch  Criteria=u2 ~= 0  Threshold=0.5
  VOLTAGE FAULT DETECTION LOGIC : Subsystem
  Vbus : Outport
  i_MAIN : Outport  Port=2
  i_APU : Outport  Port=3
  i_GND : Outport  Port=4
  i_AUX : Outport  Port=5
  wires:
  Memory1/1 -> Data Type Conversion/1
  Logical Operator/1 -> Switch4/2
  MATLAB Fcn/1 -> Memory18/1, Logical Operator/1
  VOLTAGE FAULT DETECTION LOGIC/1(Fault Signal  (Acitve Low)) -> Memory1/1
  Memory18/1 -> Mux/3
  Sqrt/1 -> VOLTAGE FAULT DETECTION LOGIC/1(In1)
  Data Type Conversion/1 -> Mux/1
  Math Function/1 -> Sum/1
  Sum/1 -> Sqrt/1
  Constant3/1 -> Switch4/3, Mux/2
  Mux/1 -> MATLAB Fcn/1
  Select/1 -> Switch4/1
  MAIN_Gen/1 -> Multiport Switch/2
  APU_Gen/1 -> Multiport Switch/3
  GND_sup/1 -> Multiport Switch/4
  AUX_sup/1 -> Multiport Switch/5
  Multiport Switch/1 -> Vbus/1, Math Function/1
  Switch4/1 -> Multiport Switch/1, Compare To Constant2/1, Compare To Constant3/1, Compare To Constant1/1, Compare To Constant4/1
  Switch/1 -> i_MAIN/1
  Switch1/1 -> i_APU/1
  Switch2/1 -> i_GND/1
  Switch3/1 -> i_AUX/1
  i_Bus/1 -> Switch/1, Switch1/1, Switch2/1, Switch3/1
  Compare To Constant4/1 -> Switch/2
  Compare To Constant1/1 -> Switch1/2
  Compare To Constant2/1 -> Switch2/2
  Compare To Constant3/1 -> Switch3/2
  Constant/1 -> Switch3/3, Switch2/3, Switch1/3, Switch/3
